simulink model "plant"  (R2025b)
settings: Solver=VariableStepAuto  StartTime=0.0  StopTime=50.0  RelTol=1e-3
undefined symbols (not defined in the file or in its folder): Rows, tau
libraries: simulink x2, dspsigops x1, dspsrcs4 x1
settings Model: Creator=strog  LastModifiedBy=strog

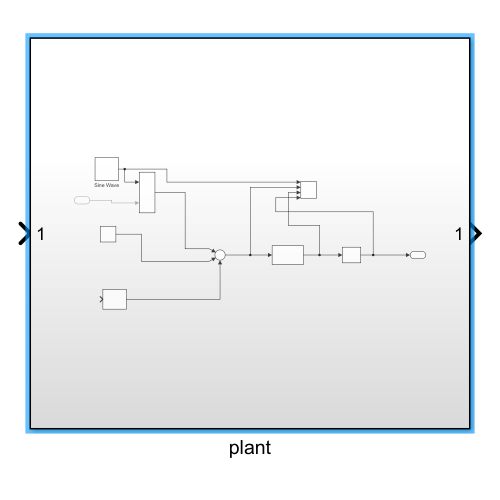
[thumbnail: Simulink's stored preview of the top-level diagram]
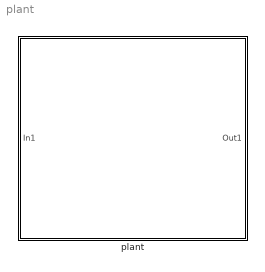
== system plant ==
  plant : Subsystem

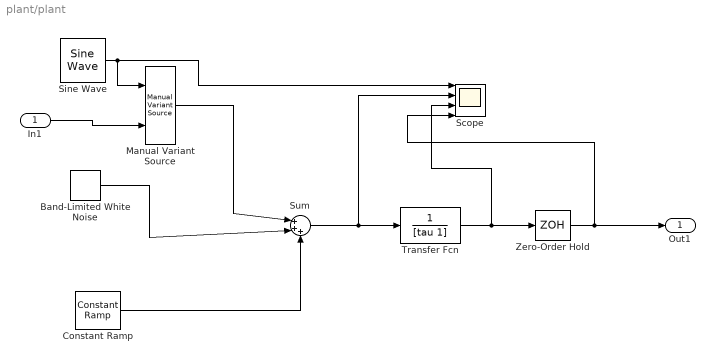
== system plant/plant ==
  In1 : Inport
  Band-Limited White Noise : simulink/Sources/Band-Limited White Noise  Cov=[0.1]  Ts=0.1  seed=[23341]
  Constant Ramp : dspsigops/Constant Ramp  L=Rows  dim=1  Slope=0.001  dataType=Same as input  isSigned=on  wordLen=16  udDataType=sfix(16)  fracBitsMode=Best precision  numFracBits=15  Offset=0
  Manual Variant Source : simulink/Signal Routing/Manual Variant Source  NumChoices=2  LabelModeActiveChoice=V_1
  Scope : Scope  NumInputPorts=4
      settings: ActiveDisplayYMinimum=-3.280270642685303  ActiveDisplayYMaximum=2.0962117324372023  DataLoggingVariableName=ScopeData2  DataLoggingSaveFormat=Array
  Sine Wave : dspsrcs4/Sine Wave  Amplitude=1  Frequency=1  Phase=0  SampleMode=Discrete  OutComplex=Real  CompMethod=Trigonometric fcn  TableSize=Speed  SampleTime=1/1000  SamplesPerFrame=1  ResetState=Restart at time zero  OutputFrames=off  dataType=double  wordLen=16  udDataType=sfix(16)  fracBitsMode=Best precision  numFracBits=15  OutDataTypeStr=double  LastOutDataTypeStr=double
  Sum : Sum  Inputs=|+++
  Transfer Fcn : TransferFcn  Denominator=[tau 1]
  Zero-Order Hold : ZeroOrderHold  SampleTime=0.01
  Out1 : Outport
  wires:
  Sine Wave/1 -> Manual Variant Source/1, Scope/1
  Band-Limited White Noise/1 -> Sum/2
  Constant Ramp/1 -> Sum/3
  Sum/1 -> Scope/2, Transfer Fcn/1
  Transfer Fcn/1 -> Scope/3, Zero-Order Hold/1
  Zero-Order Hold/1 -> Scope/4, Out1/1
  In1/1 -> Manual Variant Source/2
  Manual Variant Source/1 -> Sum/1
